simulink subsystem "Sistema_Anticolision"  (R2024b)
settings: Solver=VariableStepAuto  StartTime=0.0  StopTime=10.0  RelTol=1e-3
settings Model: Creator=Chenfu  LastModifiedBy=Chenfu

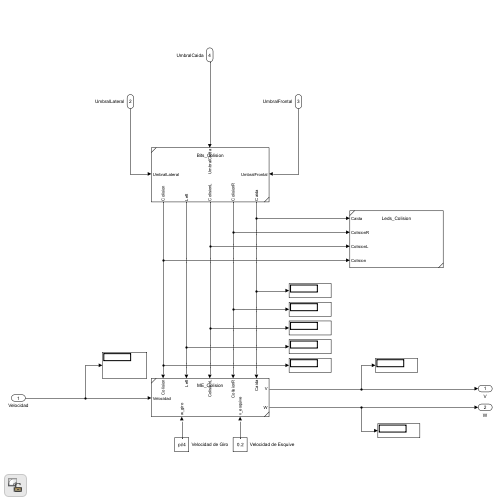
[thumbnail: Simulink's stored preview of the top-level diagram]
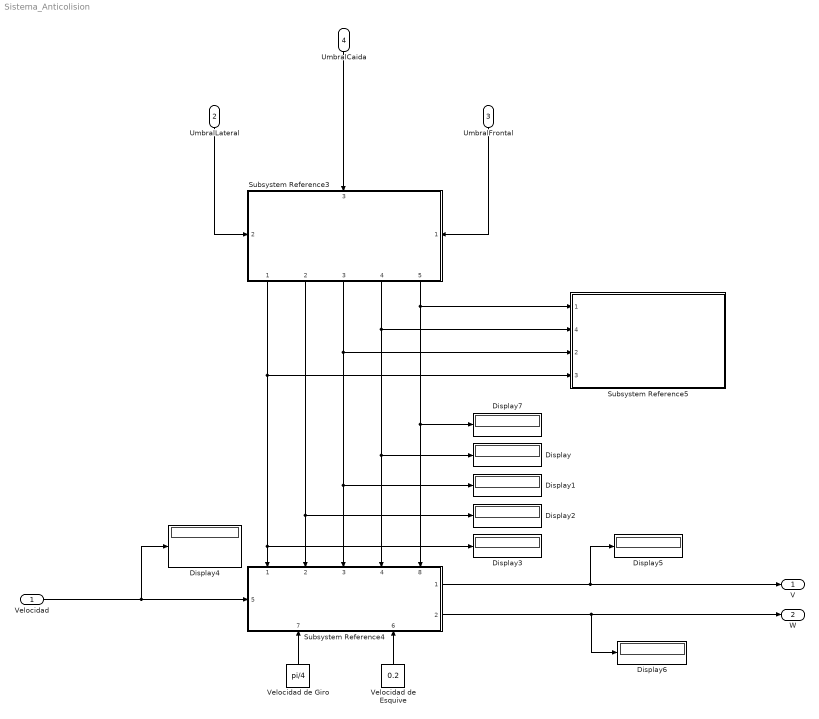
== system Sistema_Anticolision ==
  Velocidad : Inport
  UmbralLateral : Inport  Port=2
  UmbralFrontal : Inport  Port=3
  UmbralCaida : Inport  Port=4
  Display{,1..7} (8 alike) : Display
  Subsystem Reference3 : Subsystem  ReferencedSubsystem=Bits_Colision
      settings: PortSchema="{\"entries\":[{\"content\":{\"sides\":[{\"content\":{\"connectorIds\":[\"In2\"]},\"type\":\"ConnectorPlacement.EquallySpacedRectSide\",\"uuid\":\"408cd73f-1857-4da1-ae96-c05435cac705\"},{\"content\":{\"connectorIds\":[\"In1\"],\"side\":\"RIGHT\"},\"type\":\"ConnectorPlacement.EquallySpacedRectSide\",\"uuid\":\"c558c647-ecf2-46f4-93b3-68ffd7ab6733\"},{\"content\":{\"connectorIds\":[\"In3\"],\"side\":\"TOP\"},\"type\":\"ConnectorPlacement.EquallySpacedRectSide\",\"uuid\":\"d0f1560b-589e-4add-97c7-7e558b50eec2\"},{\"content\":{\"connectorIds\":[\"Out1\",\"Out2\",\"Out3\",\"Out4\",\"Out5\"],\"side\":\"BOTTOM\"},\"type\":\"ConnectorPlacement.EquallySpacedRectSide\",\"uuid\":\"e27d42a1-23f8-4a2a-9b17-20a6cb6458d1\"}]},\"type\":\"ConnectorPlacement.EquallySpacedConnector\",\"uuid\":\"6a4a7c7e-833b-4492-9d12-ab73c24b9d4d\"}],\"packageUris\":[\"http://schema.mathworks.com/mf0/Connector/R2020b\"],\"version\":\"1.0\"}"
  Subsystem Reference4 : Subsystem  ReferencedSubsystem=ME_Colision
      settings: PortSchema="{\"entries\":[{\"content\":{\"sides\":[{\"content\":{\"connectorIds\":[\"In5\"]},\"type\":\"ConnectorPlacement.EquallySpacedRectSide\",\"uuid\":\"fd240e3c-6394-4405-8519-0479f77d2d36\"},{\"content\":{\"connectorIds\":[\"Out1\",\"Out2\"],\"side\":\"RIGHT\"},\"type\":\"ConnectorPlacement.EquallySpacedRectSide\",\"uuid\":\"6add68b4-b4ce-48ef-b5c5-69d1ef184884\"},{\"content\":{\"connectorIds\":[\"In1\",\"In2\",\"In3\",\"In4\",\"In8\"],\"side\":\"TOP\"},\"type\":\"ConnectorPlacement.EquallySpacedRectSide\",\"uuid\":\"65e91425-4ef2-48e9-b7a9-d3b65ea8e822\"},{\"content\":{\"connectorIds\":[\"In7\",\"In6\"],\"side\":\"BOTTOM\"},\"type\":\"ConnectorPlacement.EquallySpacedRectSide\",\"uuid\":\"6a9c56c5-dfed-4d72-bc8b-a85f8cbcc4c7\"}]},\"type\":\"ConnectorPlacement.EquallySpacedConnector\",\"uuid\":\"4936f7de-35b8-4d13-b291-96fbfb671eec\"}],\"packageUris\":[\"http://schema.mathworks.com/mf0/Connector/R2020b\"],\"version\":\"1.0\"}"
  Subsystem Reference5 : Subsystem  ReferencedSubsystem=Leds_Colision
      settings: PortSchema="{\"entries\":[{\"content\":{\"sides\":[{\"content\":{\"connectorIds\":[\"In1\",\"In4\",\"In2\",\"In3\"]},\"type\":\"ConnectorPlacement.EquallySpacedRectSide\",\"uuid\":\"2ab864bd-d6e7-40b3-8a56-6137a7d8898f\"},{\"content\":{\"side\":\"RIGHT\"},\"type\":\"ConnectorPlacement.EquallySpacedRectSide\",\"uuid\":\"49c79b2a-2a5d-4db9-a50c-9046a80f2f2e\"},{\"content\":{\"side\":\"TOP\"},\"type\":\"ConnectorPlacement.EquallySpacedRectSide\",\"uuid\":\"55fca8d4-aafa-46b9-b77a-1d547d5b0da6\"}]},\"type\":\"ConnectorPlacement.EquallySpacedConnector\",\"uuid\":\"fa4ca95c-158a-438b-be49-b5349e28a301\"}],\"packageUris\":[\"http://schema.mathworks.com/mf0/Connector/R2020b\"],\"version\":\"1.0\"}"
  Velocidad de Esquive : Constant  Value=0.2
  Velocidad de Giro : Constant  Value=pi/4
  V : Outport
  W : Outport  Port=2
  wires:
  Subsystem Reference3/1 -> Subsystem Reference4/1, Display3/1, Subsystem Reference5/3
  Velocidad de Esquive/1 -> Subsystem Reference4/6
  Subsystem Reference3/2 -> Subsystem Reference4/2, Display2/1
  Subsystem Reference3/3 -> Subsystem Reference4/3, Display1/1, Subsystem Reference5/2
  Velocidad de Giro/1 -> Subsystem Reference4/7
  Velocidad/1 -> Subsystem Reference4/5, Display4/1
  Subsystem Reference4/1 -> V/1, Display5/1
  Subsystem Reference4/2 -> W/1, Display6/1
  UmbralLateral/1 -> Subsystem Reference3/2
  UmbralFrontal/1 -> Subsystem Reference3/1
  UmbralCaida/1 -> Subsystem Reference3/3
  Subsystem Reference3/5 -> Subsystem Reference4/8, Display7/1, Subsystem Reference5/1
  Subsystem Reference3/4 -> Subsystem Reference4/4, Display/1, Subsystem Reference5/4
